simulink model "speed"  (R2022b)
settings: Solver=VariableStepAuto  StartTime=0.0  StopTime=30  RelTol=1e-3
values from neighbouring files (symbols this model uses):
  Caf = 460    [trqvparameter.m]
  Car = 440    [trqvparameter.m]
  dwf = 1.2    [trqvparameter.m]
  Iz = 105    [trqvparameter.m]
  Ki = 5    [trqvparameter.m]
  Kp = 20    [trqvparameter.m]
  Ldwf = 1.2    [trqvparameter.m]
  Ldwr = 1.16    [trqvparameter.m]
  lf = 0.761    [trqvparameter.m]
  lr = 0.831    [trqvparameter.m]
  m = 340    [trqvparameter.m]
  Rt = 0.2    [trqvparameter.m]
libraries: simulink x19, Solver_SF x1
settings Model: Creator=12045  LastModifiedBy=12045
settings DebuggingCC: ParameterPrecisionLossMsg=none

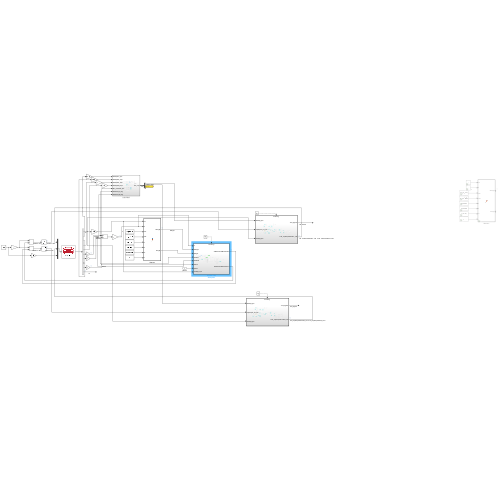
[thumbnail: Simulink's stored preview of the top-level diagram]
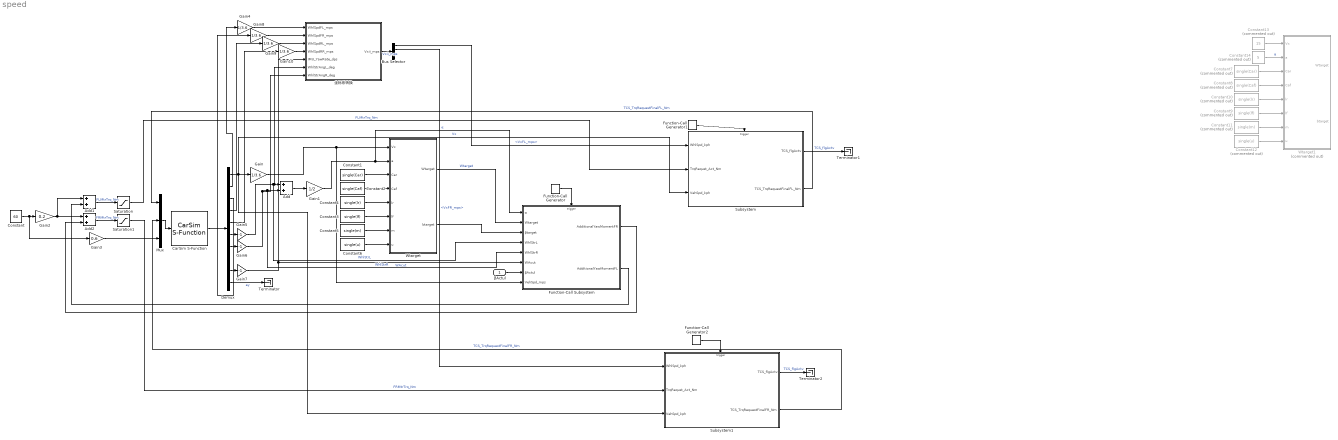
== system speed ==
  βActul : Inport
  Add : Sum
  Add1 : Sum
  Add2 : Sum
  Bus Selector : BusSelector  OutputSignals=VxFL_mps,VxFR_mps,VxRL_mps,VxRR_mps
  CarSim S-Function : Solver_SF/CarSim S-Function  Priority=1  SIMFILE=simfile.sim  Run_RTs=off  vs_state_ind=Run  StopMode_ind=Vehicle Model
  Constant : Constant  Value=60
  Constant1 : Constant  Value=single(Car)
  Constant10 : Constant  Commented=on  Value=single(lr)
  Constant11 : Constant  Commented=on  Value=single(m)
  Constant12 : Constant  Commented=on  Value=single(u)
  Constant13 : Constant  Commented=on  Value=15
  Constant14 : Constant  Commented=on  Value=5
  Constant2 : Constant  Value=single(Caf)
  Constant3 : Constant  Value=single(lf)
  Constant4 : Constant  Value=single(lr)
  Constant5 : Constant  Value=single(m)
  Constant6 : Constant  Value=single(u)
  Constant7 : Constant  Commented=on  Value=single(Car)
  Constant8 : Constant  Commented=on  Value=single(Caf)
  Constant9 : Constant  Commented=on  Value=single(lf)
  Demux : Demux  Outputs=10
  Function-Call Generator : simulink/Ports & Subsystems/Function-Call Generator  sample_time=0.01  numberOfIterations=1  DisallowWideOutput=off
  Function-Call Generator1 : simulink/Ports & Subsystems/Function-Call Generator  sample_time=0.01  numberOfIterations=1  DisallowWideOutput=off
  Function-Call Generator2 : simulink/Ports & Subsystems/Function-Call Generator  sample_time=0.01  numberOfIterations=1  DisallowWideOutput=off
  Function-Call Subsystem : Subsystem  TreatAsAtomicUnit=on
  Gain{,4,8..10} (5 alike) : Gain  Gain=1/3.6
  Gain1 : Gain  Gain=1/2
  Gain2 : Gain  Gain=0.2
  Gain3 : Gain  Gain=0.6
  Gain5 : Gain  Gain=-1
  Gain6 : Gain  Gain=-1
  Gain7 : Gain  Gain=-1
  Mux : Mux  Inputs=3
  Saturation : Saturate  UpperLimit=inf  LowerLimit=0
  Saturation1 : Saturate  UpperLimit=inf  LowerLimit=0
  Subsystem : Subsystem
  Subsystem1 : Subsystem
  Terminator : Terminator
  Terminator1 : Terminator
  Terminator2 : Terminator
  Wtarget : MATLAB Function  TreatAsAtomicUnit=on
  Wtarget1 : MATLAB Function  Commented=on  TreatAsAtomicUnit=on
  坐标系转换 : Subsystem
  wires:
  Gain1/1 -> Function-Call Subsystem/1(α), Wtarget/2(a)  "α"
  Demux/1 -> Subsystem1/3(VehSpd_kph), Subsystem/3(VehSpd_kph), Gain/1  "Vx"
  Function-Call Generator/1 -> Function-Call Subsystem/Trigger
  Wtarget/1(Wtarget) -> Function-Call Subsystem/2(Wtarget)  "Wtarget"
  Wtarget/2(btarget) -> Function-Call Subsystem/3(βtarget)
  Demux/9 -> Gain7/1
  βActul/1 -> Function-Call Subsystem/7(βActul)
  Function-Call Subsystem/1(AdditionalYawMomentFR) -> Add2/2
  CarSim S-Function/1 -> Demux/1
  Demux/6 -> Gain5/1
  Demux/7 -> Gain6/1
  Add/1 -> Gain1/1
  Gain7/1 -> 坐标系转换/5(IMU_YawRate_dps), Function-Call Subsystem/6(WAcut)  "WAcut"
  Mux/1 -> CarSim S-Function/1
  Constant/1 -> Gain3/1, Gain2/1
  Gain3/1 -> Mux/3
  Add1/1 -> Saturation/1  "FLMtrTrq_Nm"
  Add2/1 -> Saturation1/1  "FRMtrTrq_Nm"
  Gain2/1 -> Add1/1, Add2/1
  Saturation/1 -> Subsystem/2(TrqRequst_Act_Nm)  "FLMtrTrq_Nm"
  Saturation1/1 -> Subsystem1/2(TrqRequst_Act_Nm)  "FRMtrTrq_Nm"
  Gain5/1 -> 坐标系转换/6(WhlStrAngL_deg), Add/1, Function-Call Subsystem/4(WhlStrL)  "WhlStrL"
  Gain6/1 -> 坐标系转换/7(WhlStrAngR_deg), Add/2, Function-Call Subsystem/5(WhlStrR)  "WhlStrR"
  Gain/1 -> Function-Call Subsystem/8(VehSpd_mps), Wtarget/1(Vx)
  Constant5/1 -> Wtarget/7(m)
  Constant6/1 -> Wtarget/8(u)
  Constant4/1 -> Wtarget/5(lr)
  Constant2/1 -> Wtarget/4(Caf)
  Constant1/1 -> Wtarget/3(Car)
  Constant3/1 -> Wtarget/6(lf)
  Constant9/1 -> Wtarget1/6(lf)
  Constant7/1 -> Wtarget1/3(Car)
  Constant8/1 -> Wtarget1/4(Caf)
  Constant10/1 -> Wtarget1/5(lr)
  Constant12/1 -> Wtarget1/8(u)
  Constant11/1 -> Wtarget1/7(m)
  Constant13/1 -> Wtarget1/1(Vx)
  Constant14/1 -> Wtarget1/2(a)  "α"
  Function-Call Subsystem/2(AdditionalYawMomentFL) -> Add1/2
  Demux/10 -> Terminator/1  "ay"
  Function-Call Generator1/1 -> Subsystem/Trigger
  Demux/2 -> Gain4/1
  Subsystem/1(TCS_flgActv) -> Terminator1/1  "TCS_flgActv"
  Function-Call Generator2/1 -> Subsystem1/Trigger
  Demux/3 -> Gain8/1
  Subsystem1/1(TCS_flgActv) -> Terminator2/1  "TCS_flgActv"
  Subsystem/2(TCS_TrqRequestFinalFL_Nm) -> Mux/1  "TCS_TrqRequestFinalFL_Nm"
  Subsystem1/2(TCS_TrqRequestFinalFR_Nm) -> Mux/2  "TCS_TrqRequestFinalFR_Nm"
  Demux/4 -> Gain9/1
  Demux/5 -> Gain10/1
  Gain4/1 -> 坐标系转换/1(WhlSpdFL_mps)
  Gain8/1 -> 坐标系转换/2(WhlSpdFR_mps)
  Gain9/1 -> 坐标系转换/3(WhlSpdRL_mps)
  Gain10/1 -> 坐标系转换/4(WhlSpdRR_mps)
  坐标系转换/1(Vxii_mps) -> Bus Selector/1  "Vxii_mps"
  Bus Selector/1 -> Subsystem/1(WhlSpd_kph)  "<VxFL_mps>"
  Bus Selector/2 -> Subsystem1/1(WhlSpd_kph)  "<VxFR_mps>"

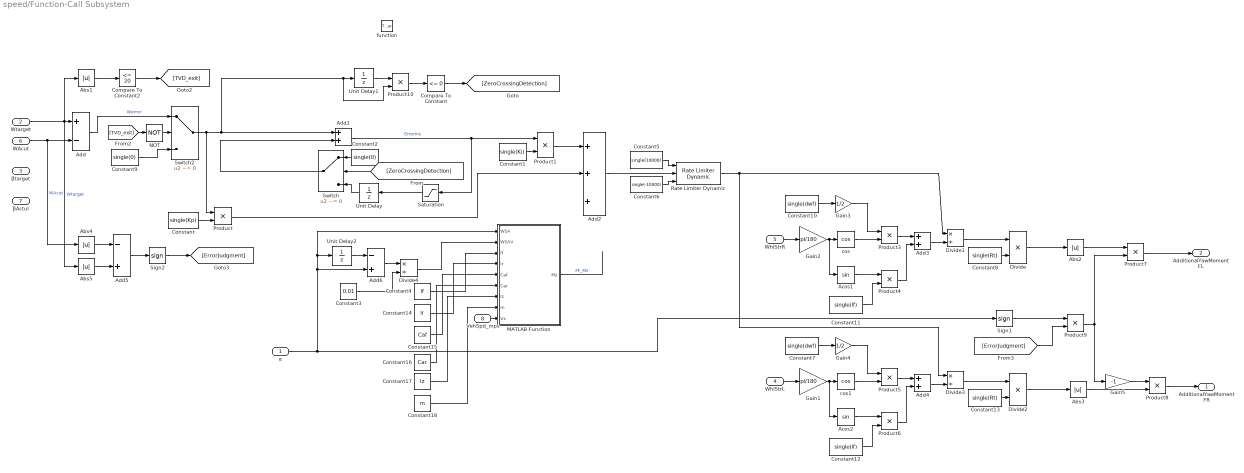
== system speed/Function-Call Subsystem ==
  α : Inport
  Wtarget : Inport  Port=2
  βtarget : Inport  Port=3
  WhlStrL : Inport  Port=4
  WhlStrR : Inport  Port=5
  WAcut : Inport  Port=6
  βActul : Inport  Port=7
  VehSpd_mps : Inport  Port=8
  function : TriggerPort  TriggerType=function-call  VariantControl=(inherit)
  Abs{1..5} (5 alike) : Abs  SaturateOnIntegerOverflow=off
  Acos1 : Trigonometry
  Acos2 : Trigonometry
  Add : Sum  Inputs=+-
  Add1 : Sum
  Add2 : Sum  Inputs=+++
  Add3 : Sum
  Add4 : Sum
  Add5 : Sum  Inputs=-+
  Add6 : Sum  Inputs=-+
  Compare To Constant : simulink/Logic and Bit Operations/Compare To Constant  relop=<=  const=0  OutDataTypeStr=boolean
  Compare To Constant2 : simulink/Logic and Bit Operations/Compare To Constant  relop=<=  const=20  OutDataTypeStr=boolean
  Constant : Constant  Value=single(Kp)
  Constant1 : Constant  Value=single(Ki)
  Constant10 : Constant  Value=single(dwf)
  Constant11 : Constant  Value=single(lf)
  Constant12 : Constant  Value=single(lf)
  Constant13 : Constant  Value=single(Rt)
  Constant14 : Constant  Value=lr
  Constant15 : Constant  Value=Caf
  Constant16 : Constant  Value=Car
  Constant17 : Constant  Value=Iz
  Constant18 : Constant  Value=m
  Constant2 : Constant  Value=single(0)
  Constant3 : Constant  Value=0.01
  Constant4 : Constant  Value=lf
  Constant5 : Constant  Value=single(10000)
  Constant6 : Constant  Value=single(-10000)
  Constant7 : Constant  Value=single(dwf)
  Constant8 : Constant  Value=single(Rt)
  Constant9 : Constant  Value=single(0)
  Divide : Product  Inputs=**
  Divide1 : Product  Inputs=*/
  Divide2 : Product  Inputs=**
  Divide3 : Product  Inputs=*/
  Divide4 : Product  Inputs=*/
  Gain1 : Gain  Gain=pi/180
  Gain2 : Gain  Gain=pi/180
  Gain3 : Gain  Gain=1/2
  Gain4 : Gain  Gain=1/2
  Gain5 : Gain  Gain=-1
  MATLAB Function : MATLAB Function  TreatAsAtomicUnit=on
  NOT : Logic  Operator=NOT  AllPortsSameDT=off  OutDataTypeStr=boolean
  Product{,1,3..10} (10 alike) : Product
  Rate Limiter Dynamic : simulink/Discontinuities/Rate Limiter Dynamic
  Saturation : Saturate  UpperLimit=10  LowerLimit=-10
  Sign1 : Signum
  Sign2 : Signum
  Switch : Switch  Criteria=u2 ~= 0  SaturateOnIntegerOverflow=off  InputSameDT=off
  Switch2 : Switch  Criteria=u2 ~= 0  SaturateOnIntegerOverflow=off  InputSameDT=off
  Unit Delay : UnitDelay  SampleTime=-1  HasFrameUpgradeWarning=on
  Unit Delay1 : UnitDelay  SampleTime=-1  HasFrameUpgradeWarning=on
  Unit Delay2 : UnitDelay  SampleTime=-1  HasFrameUpgradeWarning=on
  cos : Trigonometry  Operator=cos
  cos1 : Trigonometry  Operator=cos
  AdditionalYawMomentFR : Outport
  AdditionalYawMomentFL : Outport  Port=2
  wires:
  Wtarget/1 -> Abs5/1, Abs1/1, Add/1  "Wtarget"
  WAcut/1 -> Abs4/1, Add/2  "WAcut"
  Add/1 -> Switch2/1  "Werror"
  Constant/1 -> Product/2
  Add1/1 -> Saturation/1, Product1/1  "ErrorIns"
  Constant1/1 -> Product1/2
  Product1/1 -> Add2/1
  Product/1 -> Add2/2
  Saturation/1 -> Unit Delay/1
  Switch/1 -> Add1/2
  Constant2/1 -> Switch/1
  Unit Delay/1 -> Switch/3
  Compare To Constant/1 -> [ZeroCrossingDetection]
  [ZeroCrossingDetection] -> Switch/2
  MATLAB Function/1(Mz) -> ?  "FF_Mz"
  Constant8/1 -> Divide/2
  Constant5/1 -> Rate Limiter Dynamic/1
  Constant6/1 -> Rate Limiter Dynamic/3
  Abs1/1 -> Compare To Constant2/1
  Compare To Constant2/1 -> [TVD_exit]
  Switch2/1 -> Product10/2, Unit Delay1/1, Add1/1, Product/1
  [TVD_exit] -> NOT/1
  NOT/1 -> Switch2/2
  Constant9/1 -> Switch2/3
  WhlStrR/1 -> Gain2/1
  Gain2/1 -> Acos1/1, cos/1
  Constant10/1 -> Gain3/1
  cos/1 -> Product3/2
  Gain3/1 -> Product3/1
  Product3/1 -> Add3/1
  Acos1/1 -> Product4/1
  Constant11/1 -> Product4/2
  Product4/1 -> Add3/2
  Add3/1 -> Divide1/2
  Divide1/1 -> Divide/1
  Divide/1 -> Abs2/1
  Divide3/1 -> Divide2/1
  Add4/1 -> Divide3/2
  Product6/1 -> Add4/2
  Constant12/1 -> Product6/2
  Acos2/1 -> Product6/1
  Product5/1 -> Add4/1
  Gain4/1 -> Product5/1
  cos1/1 -> Product5/2
  Constant7/1 -> Gain4/1
  Gain1/1 -> cos1/1, Acos2/1
  WhlStrL/1 -> Gain1/1
  Rate Limiter Dynamic/1 -> Divide3/1, Divide1/1
  Constant13/1 -> Divide2/2
  Divide2/1 -> Abs3/1
  Product7/1 -> AdditionalYawMomentFL/1
  Product8/1 -> AdditionalYawMomentFR/1
  Add2/1 -> Rate Limiter Dynamic/2
  Abs2/1 -> Product7/1
  Abs3/1 -> Product8/2
  Sign2/1 -> [ErrorJudgment]
  [ErrorJudgment] -> Product9/2
  Sign1/1 -> Product9/1
  Product9/1 -> Product7/2, Gain5/1
  Gain5/1 -> Product8/1
  Abs4/1 -> Add5/1
  Abs5/1 -> Add5/2
  Add5/1 -> Sign2/1
  α/1 -> Sign1/1, MATLAB Function/1(WSA), Unit Delay2/1, Add6/2
  Unit Delay1/1 -> Product10/1
  Product10/1 -> Compare To Constant/1
  Unit Delay2/1 -> Add6/1
  Add6/1 -> Divide4/1
  Constant3/1 -> Divide4/2
  Divide4/1 -> MATLAB Function/2(WSAV)
  Constant4/1 -> MATLAB Function/3(lf)
  Constant14/1 -> MATLAB Function/4(lr)
  Constant15/1 -> MATLAB Function/5(Caf)
  Constant16/1 -> MATLAB Function/6(Car)
  Constant17/1 -> MATLAB Function/7(Iz)
  Constant18/1 -> MATLAB Function/8(m)
  VehSpd_mps/1 -> MATLAB Function/9(Vx)

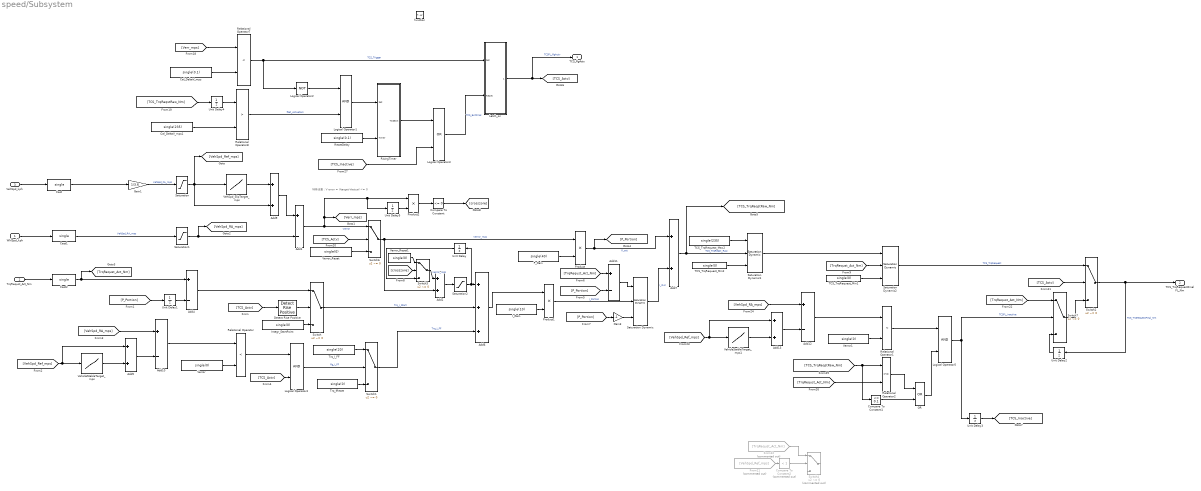
== system speed/Subsystem ==
  note: 特殊设置：V error = Vtarget-Vactual <= 0
  WhlSpd_kph : Inport
  TrqRequst_Act_Nm : Inport  Port=2
  VehSpd_kph : Inport  Port=3
  function : TriggerPort  TriggerType=function-call  VariantControl=(inherit)
  Add{1,4,10..12} (5 alike) : Sum  Inputs=+-
  Add{2,5,7,9,13} (5 alike) : Sum
  Add6 : Sum  Inputs=+++
  Cal_DeltaV_mps : Constant  Value=single(0.1)
  Cal_DeltaV_mps1 : Constant  Value=single(235)
  Cast : DataTypeConversion  OutDataTypeStr=single  SaturateOnIntegerOverflow=off  RndMeth=Floor
  Cast1 : DataTypeConversion  OutDataTypeStr=single  SaturateOnIntegerOverflow=off  RndMeth=Floor
  Cast2 : DataTypeConversion  OutDataTypeStr=single  SaturateOnIntegerOverflow=off  RndMeth=Floor
  Compare To Constant : simulink/Logic and Bit Operations/Compare To Constant  relop=<=  const=0  OutDataTypeStr=boolean
  Compare To Constant1 : simulink/Logic and Bit Operations/Compare To Constant  relop=<=  const=0.1  OutDataTypeStr=boolean
  Compare To Constant2 : simulink/Logic and Bit Operations/Compare To Constant  Commented=on  relop=<  const=1  OutDataTypeStr=boolean
  Detect Rise Positive : simulink/Logic and Bit Operations/Detect Rise Positive  vinit=0  OutDataTypeStr=boolean
  From11 : From  Commented=on  GotoTag=VehSpd_Ref_mps
  From12 : From  Commented=on  GotoTag=TrqRequst_Act_Nm
  Gain1 : Gain  Gain=1/3.6
  Gain3 : Gain  Gain=-1
  I_Gain : Constant  Value=single(10)
  Integr_StartPoint : Constant  Value=single(0)
  Latch_on : Subsystem
  Logical Operator1 : Logic  AllPortsSameDT=off  OutDataTypeStr=boolean
  Logical Operator2 : Logic  Operator=NOT  AllPortsSameDT=off  OutDataTypeStr=boolean
  Logical Operator3 : Logic  Operator=OR  AllPortsSameDT=off  OutDataTypeStr=boolean
  Logical Operator4 : Logic  AllPortsSameDT=off  OutDataTypeStr=boolean
  Logical Operator5 : Logic  AllPortsSameDT=off  OutDataTypeStr=boolean
  OR : Logic  Operator=OR  AllPortsSameDT=off  OutDataTypeStr=boolean
  P_Gain : Constant  Value=single(40)
  Product : Product
  Product1 : Product
  Product2 : Product
  Relational Operator : RelationalOperator  Operator=<  OutDataTypeStr=boolean  RndMeth=Simplest  InputSameDT=off
  Relational Operator1 : RelationalOperator  Operator=<  OutDataTypeStr=boolean  RndMeth=Simplest  InputSameDT=off
  Relational Operator2 : RelationalOperator  OutDataTypeStr=boolean  RndMeth=Simplest  InputSameDT=off
  Relational Operator7 : RelationalOperator  Operator=<  OutDataTypeStr=boolean  RndMeth=Simplest  InputSameDT=off
  Relational Operator8 : RelationalOperator  Operator=>  OutDataTypeStr=boolean  RndMeth=Simplest  InputSameDT=off
  ResetDelay : Constant  Value=single(0.1)
  RisingTimer : Subsystem
  Saturation : Saturate  UpperLimit=40  LowerLimit=0
  Saturation Dynamic : simulink/Discontinuities/Saturation Dynamic  OutMin=[]  OutMax=[]  OutDataTypeStr=Inherit: Same as second input  OutDataType=fixdt(1, 16)  OutScaling=2^-10  DoSatur=off
  Saturation Dynamic1 : simulink/Discontinuities/Saturation Dynamic  OutMin=[]  OutMax=[]  OutDataTypeStr=Inherit: Same as second input  OutDataType=fixdt(1, 16)  OutScaling=2^-10  DoSatur=off
  Saturation Dynamic2 : simulink/Discontinuities/Saturation Dynamic  OutMin=[]  OutMax=[]  OutDataTypeStr=Inherit: Same as second input  OutDataType=fixdt(1, 16)  OutScaling=2^-10  DoSatur=off
  Saturation1 : Saturate  UpperLimit=50  LowerLimit=0
  Saturation2 : Saturate  UpperLimit=400  LowerLimit=-100
  Switch{,1..3,6..7} (6 alike) : Switch  Criteria=u2 ~= 0  SaturateOnIntegerOverflow=off  InputSameDT=off
  Switch4 : Switch  Commented=on  Criteria=u2 ~= 0  SaturateOnIntegerOverflow=off  InputSameDT=off
  TCS_TrqRequest_Max2 : Constant  Value=single(235)
  TCS_TrqRequest_Min1 : Constant  Value=single(0)
  TCS_TrqRequest_Min2 : Constant  Value=single(0)
  Trq_IReset : Constant  Value=single(0)
  Trq_I_FF : Constant  Value=single(20)
  Unit Delay{,1..5} (6 alike) : UnitDelay  SampleTime=-1  HasFrameUpgradeWarning=on
  VehSpd_SlipTarget_mps : Lookup_n-D  NumberOfTableDimensions=1  BreakpointsForDimension1=[0 3 25 30]  Table=[0.2 0.2 2.5 2.5]  ExtrapMethod=Clip  InternalRulePriority=Speed  RndMeth=Simplest
  VehicleStableTarget_mps : Lookup_n-D  NumberOfTableDimensions=1  BreakpointsForDimension1=[0,3,25,30]  Table=[0.4,0.4,1.2,1.2]  ExtrapMethod=Clip  InternalRulePriority=Speed  RndMeth=Simplest
  VehicleStableTarget_mps1 : Lookup_n-D  NumberOfTableDimensions=1  BreakpointsForDimension1=[0,3,25,30]  Table=[0.4,0.4,1.2,1.2]  ExtrapMethod=Clip  InternalRulePriority=Speed  RndMeth=Simplest
  Verror : Constant  Value=single(0)
  Verror1 : Constant  Value=single(0)
  Verror_Reset : Constant  Value=single(0)
  Verror_Reset1 : Constant  Value=single(0)
  TCS_flgActv : Outport
  TCS_TrqRequestFinalFL_Nm : Outport  Port=2
  wires:
  TCS_TrqRequest_Max2/1 -> Saturation Dynamic1/1
  [TCS_Actv] -> Switch2/2
  [TrqRequst_Act_Nm] -> Switch7/1
  [VehSpd_Ref_mps] -> VehicleStableTarget_mps1/1, Add13/1
  Integr_StartPoint/1 -> Switch/3
  VehicleStableTarget_mps1/1 -> Add13/2
  [VehSpd_Ref_mps] -> Add5/1, VehicleStableTarget_mps/1
  [VehSpd_RA_mps] -> Add12/1
  [TCS_Actv] -> Switch6/2
  Cast1/1 -> Saturation1/1  "VehSpd_RA_mps"
  [TCS_Actv] -> Detect Rise Positive/1
  Saturation Dynamic1/1 -> Saturation Dynamic2/1
  Logical Operator3/1 -> Latch_on/2(Reset)  "TCS_ExitFinal"
  ResetDelay/1 -> RisingTimer/2(Timer)
  Latch_on/1(flg_TCSActv) -> TCS_flgActv/1, [TCS_Actv]  "TCSFL_flgActv"
  Unit Delay4/1 -> Relational Operator8/1
  WhlSpd_kph/1 -> Cast1/1
  Relational Operator1/1 -> Logical Operator5/1
  Product/1 -> [P_Portion], Add7/1  "P_out"
  Relational Operator7/1 -> Latch_on/1(Set), Logical Operator2/1  "TCS_Trigger"
  Switch/1 -> Add6/2  "Trq_I_Start"
  Trq_I_FF/1 -> Switch1/1
  Add13/1 -> Add12/2
  [TrqRequst_Act_Nm] -> Relational Operator2/2
  Add2/1 -> Saturation2/1
  TCS_TrqRequest_Min2/1 -> Saturation Dynamic1/3
  Add4/1 -> Switch/1
  [TCS_Inactive] -> Logical Operator3/2
  Add10/1 -> Relational Operator/1
  VehicleStableTarget_mps/1 -> Add5/2
  TrqRequst_Act_Nm/1 -> Cast2/1
  [P_Portion] -> Gain3/1
  Gain1/1 -> Saturation/1  "VehSpd_FA_mps"
  Saturation1/1 -> Add1/2, [VehSpd_RA_mps]
  Product1/1 -> Saturation Dynamic/2  "I_Portion"
  Logical Operator5/1 -> Unit Delay3/1, Switch7/2  "TCSFL_Inactive"
  Cal_DeltaV_mps1/1 -> Relational Operator8/2
  Add11/1 -> Saturation Dynamic/1
  Unit Delay3/1 -> [TCS_Inactive]
  Logical Operator1/1 -> RisingTimer/1(Set)
  [P_Portion] -> Add11/2
  Switch2/1 -> Unit Delay2/1, TCS_TrqRequestFinalFL_Nm/1  "TCS_TrqRequestFinal_Nm"
  [TCS_TrqReqstRaw_Nm] -> Compare To Constant1/1, Relational Operator2/1
  Switch1/1 -> Add6/3  "Trq_I_FF"
  [VehSpd_RA_mps] -> Add10/1
  Unit Delay/1 -> Switch3/3
  Logical Operator2/1 -> Logical Operator1/1
  Trq_IReset/1 -> Switch1/3
  Verror1/1 -> Relational Operator1/2
  Relational Operator2/1 -> OR/1
  Switch7/1 -> Switch2/3
  Add12/1 -> Relational Operator1/1
  [P_Portion] -> Unit Delay1/1
  Unit Delay1/1 -> Add4/2
  Verror/1 -> Relational Operator/2
  Saturation Dynamic2/1 -> Switch2/1  "TCS_TrqRequest"
  [TrqRequst_Act_Nm] -> Saturation Dynamic2/2
  [TrqRequst_Act_Nm] -> Add11/1
  I_Gain/1 -> Product1/2
  Switch6/1 -> Product/1, Add2/2  "Verror_mps"
  Add9/1 -> Add1/1
  VehSpd_SlipTarget_mps/1 -> Add9/1
  [TCS_TrqReqstRaw_Nm] -> Unit Delay4/1
  Add5/1 -> Add10/2
  Saturation2/1 -> Unit Delay/1, Add6/1
  Add1/1 -> Switch6/1, Unit Delay5/1, Product2/1, [Verr_mps]  "Verror"
  Verror_Reset/1 -> Switch6/3
  TCS_TrqRequest_Min1/1 -> Saturation Dynamic2/3
  Add7/1 -> Saturation Dynamic1/2, [TCS_TrqReqstRaw_Nm]  "TCS_TrqReqst_Raw"
  [Verr_mps] -> Relational Operator7/1
  Cal_DeltaV_mps/1 -> Relational Operator7/2
  Add6/1 -> Product1/1
  Relational Operator8/1 -> Logical Operator1/2  "fSat_Actuators"
  Relational Operator/1 -> Logical Operator4/1
  Saturation/1 -> Add9/2, VehSpd_SlipTarget_mps/1, [VehSpd_Ref_mps]
  P_Gain/1 -> Product/2
  Detect Rise Positive/1 -> Switch/2
  [TCS_Actv] -> Logical Operator4/2
  Gain3/1 -> Saturation Dynamic/3
  Logical Operator4/1 -> Switch1/2  "flg_I_FF"
  VehSpd_kph/1 -> Cast/1
  RisingTimer/1(TCSExit) -> Logical Operator3/1
  Saturation Dynamic/1 -> Add7/2  "I_Out"
  Cast/1 -> Gain1/1
  Cast2/1 -> Add4/1, [TrqRequst_Act_Nm]
  Unit Delay5/1 -> Product2/2
  Product2/1 -> Compare To Constant/1
  Switch3/1 -> Add2/1  "Verror_mps"
  Compare To Constant/1 -> [crosszore]
  [crosszore] -> Switch3/2
  Verror_Reset1/1 -> Switch3/1
  Unit Delay2/1 -> Switch7/3
  From11/1 -> Compare To Constant2/1
  Compare To Constant2/1 -> Switch4/2
  From12/1 -> Switch4/1
  Compare To Constant1/1 -> OR/2
  OR/1 -> Logical Operator5/2

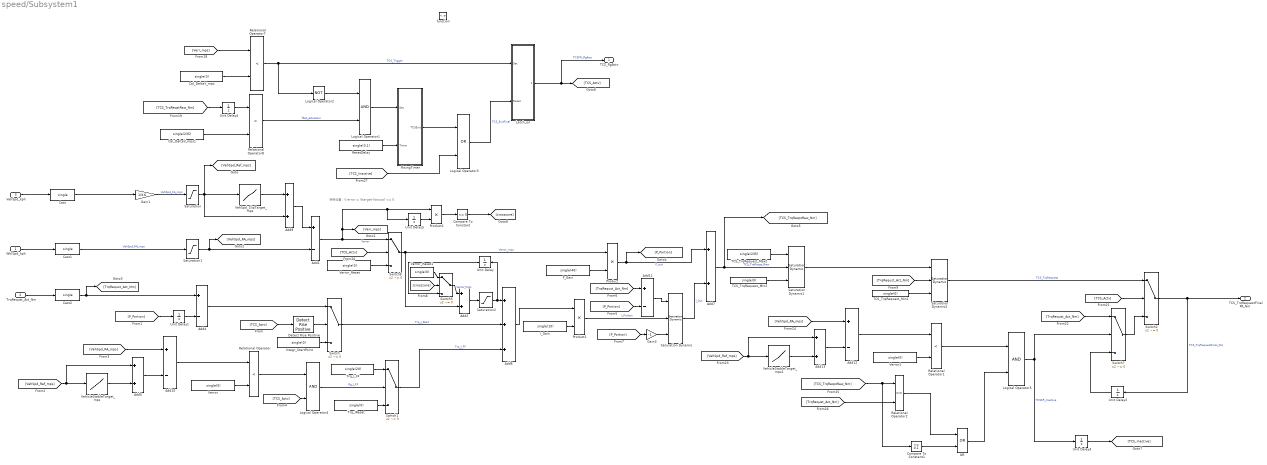
== system speed/Subsystem1 ==
  note: 特殊设置：V error = Vtarget-Vactual <= 0
  WhlSpd_kph : Inport
  TrqRequst_Act_Nm : Inport  Port=2
  VehSpd_kph : Inport  Port=3
  function : TriggerPort  TriggerType=function-call  VariantControl=(inherit)
  Add{1,4,10..12} (5 alike) : Sum  Inputs=+-
  Add{2,5,7,9,13} (5 alike) : Sum
  Add6 : Sum  Inputs=+++
  Cal_DeltaV_mps : Constant  Value=single(0)
  Cal_DeltaV_mps1 : Constant  Value=single(235)
  Cast : DataTypeConversion  OutDataTypeStr=single  SaturateOnIntegerOverflow=off  RndMeth=Floor
  Cast1 : DataTypeConversion  OutDataTypeStr=single  SaturateOnIntegerOverflow=off  RndMeth=Floor
  Cast2 : DataTypeConversion  OutDataTypeStr=single  SaturateOnIntegerOverflow=off  RndMeth=Floor
  Compare To Constant : simulink/Logic and Bit Operations/Compare To Constant  relop=<=  const=0  OutDataTypeStr=boolean
  Compare To Constant1 : simulink/Logic and Bit Operations/Compare To Constant  relop=<=  const=0.1  OutDataTypeStr=boolean
  Detect Rise Positive : simulink/Logic and Bit Operations/Detect Rise Positive  vinit=0  OutDataTypeStr=boolean
  Gain1 : Gain  Gain=1/3.6
  Gain3 : Gain  Gain=-1
  I_Gain : Constant  Value=single(10)
  Integr_StartPoint : Constant  Value=single(0)
  Latch_on : Subsystem
  Logical Operator1 : Logic  AllPortsSameDT=off  OutDataTypeStr=boolean
  Logical Operator2 : Logic  Operator=NOT  AllPortsSameDT=off  OutDataTypeStr=boolean
  Logical Operator3 : Logic  Operator=OR  AllPortsSameDT=off  OutDataTypeStr=boolean
  Logical Operator4 : Logic  AllPortsSameDT=off  OutDataTypeStr=boolean
  Logical Operator5 : Logic  AllPortsSameDT=off  OutDataTypeStr=boolean
  OR : Logic  Operator=OR  AllPortsSameDT=off  OutDataTypeStr=boolean
  P_Gain : Constant  Value=single(40)
  Product : Product
  Product1 : Product
  Product2 : Product
  Relational Operator : RelationalOperator  Operator=<  OutDataTypeStr=boolean  RndMeth=Simplest  InputSameDT=off
  Relational Operator1 : RelationalOperator  Operator=<  OutDataTypeStr=boolean  RndMeth=Simplest  InputSameDT=off
  Relational Operator2 : RelationalOperator  OutDataTypeStr=boolean  RndMeth=Simplest  InputSameDT=off
  Relational Operator7 : RelationalOperator  Operator=<  OutDataTypeStr=boolean  RndMeth=Simplest  InputSameDT=off
  Relational Operator8 : RelationalOperator  Operator=>  OutDataTypeStr=boolean  RndMeth=Simplest  InputSameDT=off
  ResetDelay : Constant  Value=single(0.1)
  RisingTimer : Subsystem
  Saturation : Saturate  UpperLimit=40  LowerLimit=0
  Saturation Dynamic : simulink/Discontinuities/Saturation Dynamic  OutMin=[]  OutMax=[]  OutDataTypeStr=Inherit: Same as second input  OutDataType=fixdt(1, 16)  OutScaling=2^-10  DoSatur=off
  Saturation Dynamic1 : simulink/Discontinuities/Saturation Dynamic  OutMin=[]  OutMax=[]  OutDataTypeStr=Inherit: Same as second input  OutDataType=fixdt(1, 16)  OutScaling=2^-10  DoSatur=off
  Saturation Dynamic2 : simulink/Discontinuities/Saturation Dynamic  OutMin=[]  OutMax=[]  OutDataTypeStr=Inherit: Same as second input  OutDataType=fixdt(1, 16)  OutScaling=2^-10  DoSatur=off
  Saturation1 : Saturate  UpperLimit=50  LowerLimit=0
  Saturation2 : Saturate  UpperLimit=400  LowerLimit=-100
  Switch{,1..3,6..7} (6 alike) : Switch  Criteria=u2 ~= 0  SaturateOnIntegerOverflow=off  InputSameDT=off
  TCS_TrqRequest_Max2 : Constant  Value=single(235)
  TCS_TrqRequest_Min1 : Constant  Value=single(0)
  TCS_TrqRequest_Min2 : Constant  Value=single(0)
  Trq_IReset : Constant  Value=single(0)
  Trq_I_FF : Constant  Value=single(20)
  Unit Delay{,1..5} (6 alike) : UnitDelay  SampleTime=-1  HasFrameUpgradeWarning=on
  VehSpd_SlipTarget_mps : Lookup_n-D  NumberOfTableDimensions=1  BreakpointsForDimension1=[0 3 25 30]  Table=[0.2 0.2 2.5 2.5]  ExtrapMethod=Clip  InternalRulePriority=Speed  RndMeth=Simplest
  VehicleStableTarget_mps : Lookup_n-D  NumberOfTableDimensions=1  BreakpointsForDimension1=[0,3,25,30]  Table=[0.4,0.4,1.2,1.2]  ExtrapMethod=Clip  InternalRulePriority=Speed  RndMeth=Simplest
  VehicleStableTarget_mps1 : Lookup_n-D  NumberOfTableDimensions=1  BreakpointsForDimension1=[0,3,25,30]  Table=[0.4,0.4,1.2,1.2]  ExtrapMethod=Clip  InternalRulePriority=Speed  RndMeth=Simplest
  Verror : Constant  Value=single(0)
  Verror1 : Constant  Value=single(0)
  Verror_Reset : Constant  Value=single(0)
  Verror_Reset1 : Constant  Value=single(0)
  TCS_flgActv : Outport
  TCS_TrqRequestFinalFR_Nm : Outport  Port=2
  wires:
  Unit Delay2/1 -> Switch7/3
  Verror_Reset1/1 -> Switch3/1
  [crosszore] -> Switch3/2
  Compare To Constant/1 -> [crosszore]
  Switch3/1 -> Add2/1  "Verror_mps"
  Product2/1 -> Compare To Constant/1
  Unit Delay5/1 -> Product2/2
  Cast2/1 -> [TrqRequst_Act_Nm], Add4/1
  Cast/1 -> Gain1/1
  Saturation Dynamic/1 -> Add7/2  "I_Out"
  RisingTimer/1(TCSExit) -> Logical Operator3/1
  VehSpd_kph/1 -> Cast/1
  Logical Operator4/1 -> Switch1/2  "flg_I_FF"
  Gain3/1 -> Saturation Dynamic/3
  [TCS_Actv] -> Logical Operator4/2
  Detect Rise Positive/1 -> Switch/2
  P_Gain/1 -> Product/2
  Saturation/1 -> VehSpd_SlipTarget_mps/1, [VehSpd_Ref_mps], Add9/2
  Relational Operator/1 -> Logical Operator4/1
  Relational Operator8/1 -> Logical Operator1/2  "fSat_Actuators"
  Add6/1 -> Product1/1
  Cal_DeltaV_mps/1 -> Relational Operator7/2
  [Verr_mps] -> Relational Operator7/1
  Add7/1 -> [TCS_TrqReqstRaw_Nm], Saturation Dynamic1/2  "TCS_TrqReqst_Raw"
  TCS_TrqRequest_Min1/1 -> Saturation Dynamic2/3
  Verror_Reset/1 -> Switch6/3
  Add1/1 -> [Verr_mps], Product2/1, Unit Delay5/1, Switch6/1  "Verror"
  Saturation2/1 -> Add6/1, Unit Delay/1
  Add5/1 -> Add10/2
  [TCS_TrqReqstRaw_Nm] -> Unit Delay4/1
  VehSpd_SlipTarget_mps/1 -> Add9/1
  Add9/1 -> Add1/1
  Switch6/1 -> Add2/2, Product/1  "Verror_mps"
  I_Gain/1 -> Product1/2
  [TrqRequst_Act_Nm] -> Add11/1
  [TrqRequst_Act_Nm] -> Saturation Dynamic2/2
  Saturation Dynamic2/1 -> Switch2/1  "TCS_TrqRequest"
  Verror/1 -> Relational Operator/2
  Unit Delay1/1 -> Add4/2
  [P_Portion] -> Unit Delay1/1
  Add12/1 -> Relational Operator1/1
  Switch7/1 -> Switch2/3
  Relational Operator2/1 -> OR/1
  Verror1/1 -> Relational Operator1/2
  Trq_IReset/1 -> Switch1/3
  Logical Operator2/1 -> Logical Operator1/1
  Unit Delay/1 -> Switch3/3
  [VehSpd_RA_mps] -> Add10/1
  Switch1/1 -> Add6/3  "Trq_I_FF"
  Switch2/1 -> TCS_TrqRequestFinalFR_Nm/1, Unit Delay2/1  "TCS_TrqRequestFinal_Nm"
  [P_Portion] -> Add11/2
  Logical Operator1/1 -> RisingTimer/1(Set)
  Unit Delay3/1 -> [TCS_Inactive]
  Add11/1 -> Saturation Dynamic/1
  Cal_DeltaV_mps1/1 -> Relational Operator8/2
  Logical Operator5/1 -> Unit Delay3/1, Switch7/2  "TCSFR_Inactive"
  Product1/1 -> Saturation Dynamic/2  "I_Portion"
  Saturation1/1 -> [VehSpd_RA_mps], Add1/2
  Gain1/1 -> Saturation/1  "VehSpd_FA_mps"
  [P_Portion] -> Gain3/1
  TrqRequst_Act_Nm/1 -> Cast2/1
  VehicleStableTarget_mps/1 -> Add5/2
  Add10/1 -> Relational Operator/1
  [TCS_Inactive] -> Logical Operator3/2
  Add4/1 -> Switch/1
  TCS_TrqRequest_Min2/1 -> Saturation Dynamic1/3
  Add2/1 -> Saturation2/1
  [TrqRequst_Act_Nm] -> Relational Operator2/2
  Add13/1 -> Add12/2
  Trq_I_FF/1 -> Switch1/1
  Switch/1 -> Add6/2  "Trq_I_Start"
  Relational Operator7/1 -> Logical Operator2/1, Latch_on/1(Set)  "TCS_Trigger"
  Product/1 -> Add7/1, [P_Portion]  "P_out"
  Relational Operator1/1 -> Logical Operator5/1
  WhlSpd_kph/1 -> Cast1/1
  Unit Delay4/1 -> Relational Operator8/1
  Latch_on/1(flg_TCSActv) -> [TCS_Actv], TCS_flgActv/1  "TCSFR_flgActv"
  ResetDelay/1 -> RisingTimer/2(Timer)
  Logical Operator3/1 -> Latch_on/2(Reset)  "TCS_ExitFinal"
  Saturation Dynamic1/1 -> Saturation Dynamic2/1
  [TCS_Actv] -> Detect Rise Positive/1
  Cast1/1 -> Saturation1/1  "VehSpd_RA_mps"
  [TCS_Actv] -> Switch6/2
  [VehSpd_RA_mps] -> Add12/1
  [VehSpd_Ref_mps] -> VehicleStableTarget_mps/1, Add5/1
  VehicleStableTarget_mps1/1 -> Add13/2
  Integr_StartPoint/1 -> Switch/3
  [VehSpd_Ref_mps] -> Add13/1, VehicleStableTarget_mps1/1
  [TrqRequst_Act_Nm] -> Switch7/1
  [TCS_Actv] -> Switch2/2
  TCS_TrqRequest_Max2/1 -> Saturation Dynamic1/1
  [TCS_TrqReqstRaw_Nm] -> Relational Operator2/1, Compare To Constant1/1
  Compare To Constant1/1 -> OR/2
  OR/1 -> Logical Operator5/2

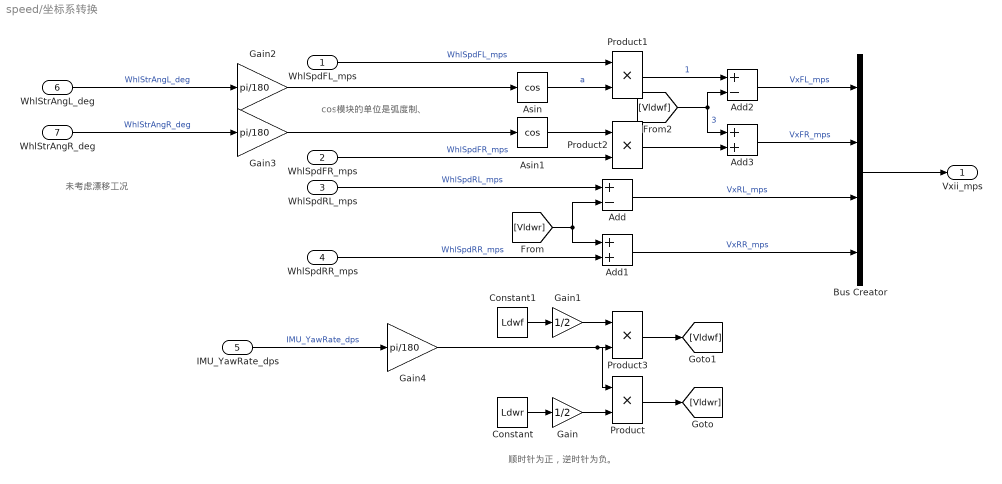
== system speed/坐标系转换 ==
  note: cos模块的单位是弧度制、
  note: 未考虑漂移工况
  note: 顺时针为正，逆时针为负。
  WhlSpdFL_mps : Inport
  WhlSpdFR_mps : Inport  Port=2
  WhlSpdRL_mps : Inport  Port=3
  WhlSpdRR_mps : Inport  Port=4
  IMU_YawRate_dps : Inport  Port=5
  WhlStrAngL_deg : Inport  Port=6
  WhlStrAngR_deg : Inport  Port=7
  Add : Sum  Inputs=+-
  Add1 : Sum
  Add2 : Sum  Inputs=+-
  Add3 : Sum
  Asin : Trigonometry  Operator=cos
  Asin1 : Trigonometry  Operator=cos
  Bus Creator : BusCreator  Inputs=4
  Constant : Constant  Value=Ldwr
  Constant1 : Constant  Value=Ldwf
  Gain : Gain  Gain=1/2
  Gain1 : Gain  Gain=1/2
  Gain2 : Gain  Gain=pi/180
  Gain3 : Gain  Gain=pi/180
  Gain4 : Gain  Gain=pi/180
  Product{,1..3} (4 alike) : Product
  Vxii_mps : Outport
  wires:
  Constant/1 -> Gain/1
  Gain/1 -> Product/2
  IMU_YawRate_dps/1 -> Gain4/1  "IMU_YawRate_dps"
  WhlSpdRL_mps/1 -> Add/1  "WhlSpdRL_mps"
  WhlSpdRR_mps/1 -> Add1/2  "WhlSpdRR_mps"
  Product/1 -> [Vldwr]
  [Vldwr] -> Add/2, Add1/1
  WhlSpdFL_mps/1 -> Product1/1  "WhlSpdFL_mps"
  WhlSpdFR_mps/1 -> Product2/2  "WhlSpdFR_mps"
  Constant1/1 -> Gain1/1
  Gain1/1 -> Product3/1
  Product3/1 -> [Vldwf]
  Product1/1 -> Add2/1  "1"
  [Vldwf] -> Add2/2, Add3/1  "3"
  Product2/1 -> Add3/2
  Add2/1 -> Bus Creator/1  "VxFL_mps"
  Add/1 -> Bus Creator/3  "VxRL_mps"
  Add3/1 -> Bus Creator/2  "VxFR_mps"
  Add1/1 -> Bus Creator/4  "VxRR_mps"
  Bus Creator/1 -> Vxii_mps/1
  Asin1/1 -> Product2/1
  WhlStrAngR_deg/1 -> Gain3/1  "WhlStrAngR_deg"
  WhlStrAngL_deg/1 -> Gain2/1  "WhlStrAngL_deg"
  Asin/1 -> Product1/2  "a"
  Gain2/1 -> Asin/1
  Gain3/1 -> Asin1/1
  Gain4/1 -> Product/1, Product3/2

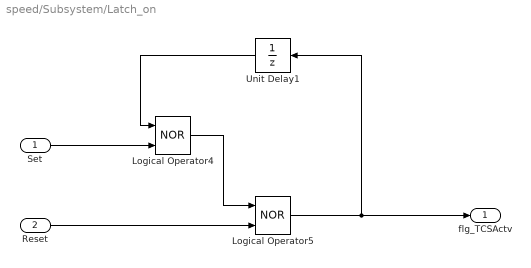
== system speed/Subsystem/Latch_on ==
  Set : Inport
  Reset : Inport  Port=2
  Logical Operator4 : Logic  Operator=NOR  AllPortsSameDT=off  OutDataTypeStr=boolean
  Logical Operator5 : Logic  Operator=NOR  AllPortsSameDT=off  OutDataTypeStr=boolean
  Unit Delay1 : UnitDelay  SampleTime=-1  HasFrameUpgradeWarning=on
  flg_TCSActv : Outport
  wires:
  Logical Operator5/1 -> flg_TCSActv/1, Unit Delay1/1
  Reset/1 -> Logical Operator5/2
  Unit Delay1/1 -> Logical Operator4/1
  Set/1 -> Logical Operator4/2
  Logical Operator4/1 -> Logical Operator5/1

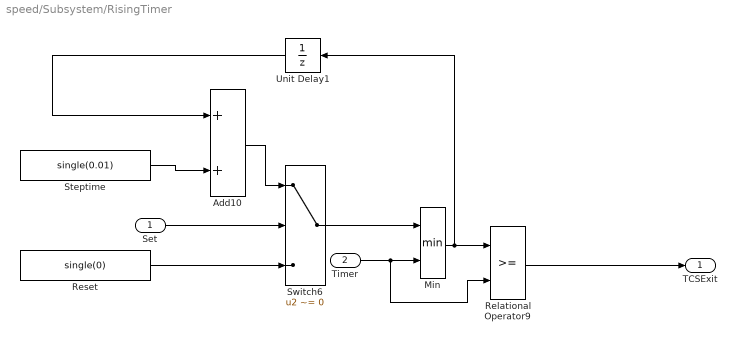
== system speed/Subsystem/RisingTimer ==
  Set : Inport
  Timer : Inport  Port=2
  Add10 : Sum
  Min : MinMax  Inputs=2
  Relational Operator9 : RelationalOperator  OutDataTypeStr=boolean  RndMeth=Simplest  InputSameDT=off
  Reset : Constant  Value=single(0)
  Steptime : Constant  Value=single(0.01)
  Switch6 : Switch  Criteria=u2 ~= 0  SaturateOnIntegerOverflow=off  InputSameDT=off
  Unit Delay1 : UnitDelay  SampleTime=-1  HasFrameUpgradeWarning=on
  TCSExit : Outport
  wires:
  Add10/1 -> Switch6/1
  Set/1 -> Switch6/2
  Min/1 -> Unit Delay1/1, Relational Operator9/1
  Unit Delay1/1 -> Add10/1
  Timer/1 -> Relational Operator9/2, Min/2
  Reset/1 -> Switch6/3
  Relational Operator9/1 -> TCSExit/1
  Steptime/1 -> Add10/2
  Switch6/1 -> Min/1

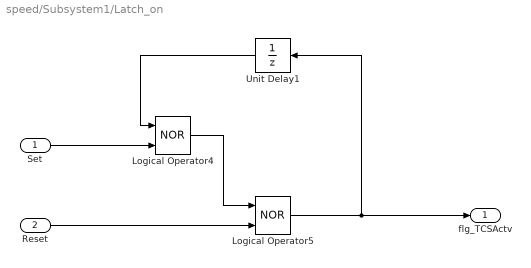
== system speed/Subsystem1/Latch_on ==
  Set : Inport
  Reset : Inport  Port=2
  Logical Operator4 : Logic  Operator=NOR  AllPortsSameDT=off  OutDataTypeStr=boolean
  Logical Operator5 : Logic  Operator=NOR  AllPortsSameDT=off  OutDataTypeStr=boolean
  Unit Delay1 : UnitDelay  SampleTime=-1  HasFrameUpgradeWarning=on
  flg_TCSActv : Outport
  wires:
  Logical Operator4/1 -> Logical Operator5/1
  Set/1 -> Logical Operator4/2
  Unit Delay1/1 -> Logical Operator4/1
  Reset/1 -> Logical Operator5/2
  Logical Operator5/1 -> Unit Delay1/1, flg_TCSActv/1

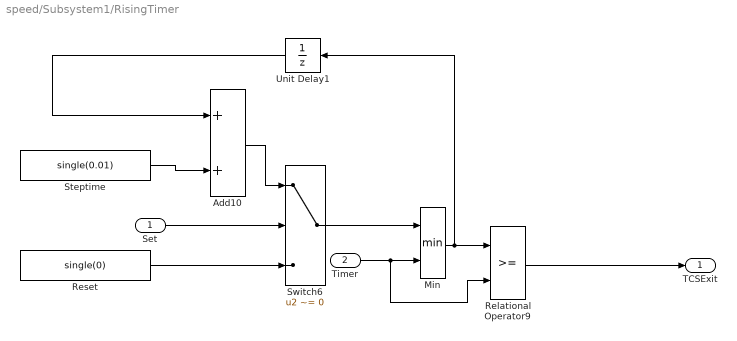
== system speed/Subsystem1/RisingTimer ==
  Set : Inport
  Timer : Inport  Port=2
  Add10 : Sum
  Min : MinMax  Inputs=2
  Relational Operator9 : RelationalOperator  OutDataTypeStr=boolean  RndMeth=Simplest  InputSameDT=off
  Reset : Constant  Value=single(0)
  Steptime : Constant  Value=single(0.01)
  Switch6 : Switch  Criteria=u2 ~= 0  SaturateOnIntegerOverflow=off  InputSameDT=off
  Unit Delay1 : UnitDelay  SampleTime=-1  HasFrameUpgradeWarning=on
  TCSExit : Outport
  wires:
  Switch6/1 -> Min/1
  Steptime/1 -> Add10/2
  Relational Operator9/1 -> TCSExit/1
  Reset/1 -> Switch6/3
  Timer/1 -> Min/2, Relational Operator9/2
  Unit Delay1/1 -> Add10/1
  Min/1 -> Relational Operator9/1, Unit Delay1/1
  Set/1 -> Switch6/2
  Add10/1 -> Switch6/1

== matlab function speed/Wtarget1 ==
  data: Vx input size=1; Wtarget output size=1; a input size=1; Car input size=1; Caf input size=1; lr input size=1; lf input size=1; m input; u input; btarget output
function [Wtarget,btarget] = fcn(Vx,a,Car,Caf,lr,lf,m,u)
Wdes = Vx*a/(lf+lr+(m*Vx*Vx*(lr*Car-lf*Caf)/(Caf*Car*(lr+lf)*2)));
Wu = 0.85*u*9.8/Vx;
if abs(Wdes)<=Wu
Wtarget = Wdes;
else
    Wtarget = Wu*sign(Wdes);
end
bdes = (lr-lf*m*Vx*Vx/Car/(lf+lr)/2)*a/(lr+lf+m*Vx*Vx*(lr*Car-lf*Caf)/Car/Caf/(lf+lr)/2);
bu = atan(0.02*u*9.8);
if abs(bdes)<=bu
btarget = bdes;
else
    btarget = bu*sign(bdes);
end

== matlab function speed/Wtarget ==
  data: Vx input size=1; Wtarget output size=1; a input size=1; Car input size=1; Caf input size=1; lr input size=1; lf input size=1; m input; u input; btarget output
function [Wtarget,btarget] = fcn(Vx,a,Car,Caf,lr,lf,m,u)
Wdes = Vx*a/(lf+lr+(m*Vx*Vx*(lr*Car-lf*Caf)/Caf/Car/(lr+lf)/2));
Wu = 0.85*u*9.8/Vx;
%if abs(Wdes)<=Wu
Wtarget = Wdes;
%else
 %   Wtarget = Wu*sign(Wdes);
%end
bdes = (lr-lf*m*Vx*Vx/Car/(lf+lr)/2)*a/(lr+lf+m*Vx*Vx*(lr*Car-lf*Caf)/Car/Caf/(lf+lr)/2);
bu = atan(0.02*u*9.8);
if abs(bdes)<=bu
btarget = bdes;
else
    btarget = bu*sign(bdes);
end

== matlab function speed/Function-Call Subsystem/MATLAB Function ==
  data: WSA input; Mz output; WSAV input; lf input; lr input; Caf input; Car input; Iz input; m input; Vx input
function Mz = fcn(WSA,WSAV,lf,lr,Caf,Car,Iz,m,Vx)

Mz = (((lf*lf*Caf+lr*lr*Car)/Iz/Vx)*(-Caf/m/Vx)-((lf*Caf-lr*Car)/m/Vx/Vx-1)*(-lf*Caf/Iz))*Iz*WSA/((lf*Caf-lr*Car)/m/Vx/Vx-1)-(-Caf/m/Vx)*Iz*WSAV/((lf*Caf-lr*Car)/m/Vx/Vx-1);
